simulink model "Accelorometer_MATLAB_Simulink"  (R2023b)
settings: Solver=FixedStepAuto  StartTime=0.0  StopTime=inf  FixedStep=0.01  RelTol=1e-3  EnableMultiTasking=on
libraries: arduinolib x3
settings Model: ExtModeTrigDuration=2  Creator=3609  LastModifiedBy=3589
settings OptimizationCC: EnhancedBackFolding=on  PassReuseOutputArgsAs=Individual arguments  ZeroExternalMemoryAtStartup=off  ZeroInternalMemoryAtStartup=off  MaxStackSize=64  OptimizeBlockOrder=speed  DifferentSizesBufferReuse=on  OptimizationCustomize=off  EfficientTunableParamExpr=on
settings DebuggingCC: ParameterTunabilityLossMsg=error
settings HardwareCC: ProdBitPerInt=16  ProdBitPerPointer=16  ProdBitPerSizeT=16  ProdBitPerPtrDiffT=16  ProdLargestAtomicFloat=None  ProdWordSize=8  ProdHWDeviceType=Atmel->AVR
settings SFSimCC: MATLABDynamicMemAlloc=off
settings RTWCC: Description=Embedded Coder  SystemTargetFile=ert.tlc  HardwareBoard=Arduino Uno  TemplateMakefile=ert_default_tmf  Toolchain=Arduino AVR  BuildConfiguration=Faster Runs
settings CodeAppCC: ForceParamTrailComments=on  IgnoreCustomStorageClasses=off  OperatorAnnotations=on  SimulinkDataObjDesc=on  SFDataObjDesc=on  InsertBlockDesc=on
settings ERTTargetCC: SupportContinuousTime=on  SupportVariableSizeSignals=on  ExtModeTransport=3  ExtModeStaticAlloc=on  ExtModeAutomaticAllocSize=off  ExtModeStaticAllocSize=250  ExtModeMexFile=ext_xcp  ExtModeIntrfLevel=Level2 - Open

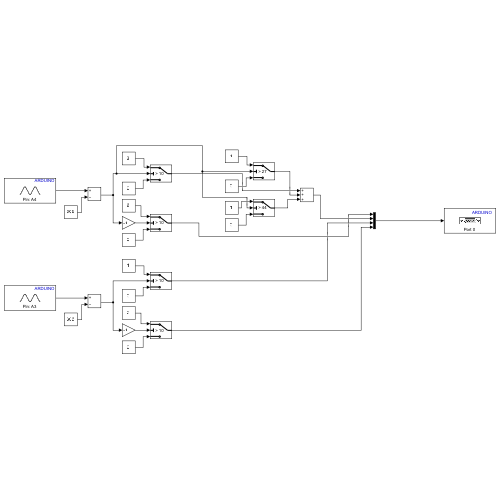
[thumbnail: Simulink's stored preview of the top-level diagram]
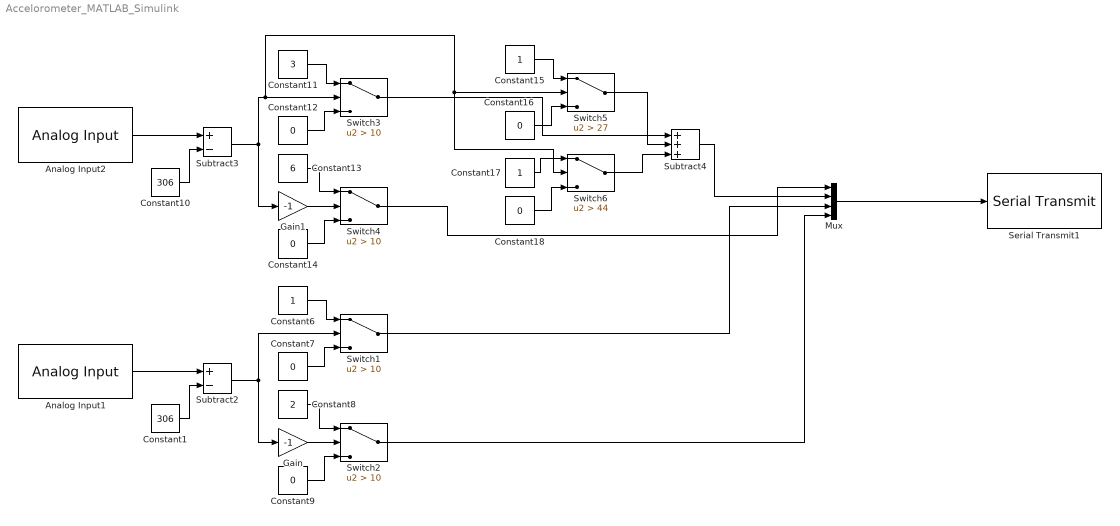
== system Accelorometer_MATLAB_Simulink ==
  Analog Input1 : arduinolib/Analog Input  pinNumber=3  ReadResultsOnly=off  ConversionTriggerSource=Software  ExternalTriggerType=uint32( 0 )  OutputDataType=uint16  EnableConversionCompleteNotify=off  EnableOuputStatus=off  SampleTime=-1  blockPlatform=arduino
  Analog Input2 : arduinolib/Analog Input  pinNumber=4  ReadResultsOnly=off  ConversionTriggerSource=Software  ExternalTriggerType=uint32( 0 )  OutputDataType=uint16  EnableConversionCompleteNotify=off  EnableOuputStatus=off  SampleTime=-1  blockPlatform=arduino
  Constant1 : Constant  Value=306
  Constant10 : Constant  Value=306
  Constant11 : Constant  Value=3
  Constant{7,9,12,14,16,18} (6 alike) : Constant  Value=0
  Constant13 : Constant  Value=6
  Constant15 : Constant
  Constant17 : Constant
  Constant6 : Constant
  Constant8 : Constant  Value=2
  Gain : Gain  Gain=-1
  Gain1 : Gain  Gain=-1
  Mux : Mux
  Serial Transmit1 : arduinolib/Serial Transmit  portNumber=0  sendmode=println  sendformat=Decimal  floatprecision=1  blockPlatform=arduino
  Subtract2 : Sum  Inputs=+-
  Subtract3 : Sum  Inputs=+-
  Subtract4 : Sum  Inputs=+++
  Switch{1..4} (4 alike) : Switch  Criteria=u2 > Threshold  Threshold=10  SaturateOnIntegerOverflow=off  InputSameDT=off
  Switch5 : Switch  Criteria=u2 > Threshold  Threshold=27  SaturateOnIntegerOverflow=off  InputSameDT=off
  Switch6 : Switch  Criteria=u2 > Threshold  Threshold=44  SaturateOnIntegerOverflow=off  InputSameDT=off
  wires:
  Constant7/1 -> Switch1/3
  Constant6/1 -> Switch1/1
  Analog Input1/1 -> Subtract2/1
  Constant1/1 -> Subtract2/2
  Subtract2/1 -> Gain/1, Switch1/2
  Gain/1 -> Switch2/2
  Constant9/1 -> Switch2/3
  Constant8/1 -> Switch2/1
  Constant14/1 -> Switch4/3
  Constant13/1 -> Switch4/1
  Gain1/1 -> Switch4/2
  Constant12/1 -> Switch3/3
  Constant11/1 -> Switch3/1
  Constant10/1 -> Subtract3/2
  Analog Input2/1 -> Subtract3/1
  Constant15/1 -> Switch5/1
  Subtract3/1 -> Gain1/1, Switch6/2, Switch5/2, Switch3/2
  Constant16/1 -> Switch5/3
  Constant18/1 -> Switch6/3
  Constant17/1 -> Switch6/1
  Switch3/1 -> Subtract4/1
  Switch5/1 -> Subtract4/2
  Switch6/1 -> Subtract4/3
  Switch4/1 -> Mux/1
  Switch1/1 -> Mux/3
  Subtract4/1 -> Mux/2
  Switch2/1 -> Mux/4
  Mux/1 -> Serial Transmit1/1
